simulink model "differential_drive"  (R2023b)
settings: Solver=VariableStepAuto  StartTime=0.0  StopTime=SimulationTime  RelTol=1e-3
values from neighbouring files (symbols this model uses):
  D_ao = 1    [gtg_ao_wf.m]
  D_wf = 1.5    [gtg_ao_wf.m]
  l = 0.5    [gtg_ao_wf.m]
  P = 10    [gtg_ao_wf.m]
  r = 0.1    [gtg_ao_wf.m]
  thetainit = 0    [gtg_ao_wf.m]
  tol = 0.1    [gtg_ao_wf.m]
  v = 0.1    [gtg_ao_wf.m]
  xg = gPos(2)    [gtg_ao_wf.m]
  xinit = sPos(2)    [gtg_ao_wf.m]
  yg = gPos(1)    [gtg_ao_wf.m]
  yinit = sPos(1)    [gtg_ao_wf.m]
undefined symbols (not defined in the file or in its folder): Z
libraries: slpidlib x1
settings Model: PauseTimes=425  PacingRate=0.100000  Creator=npn01  LastModifiedBy=Mikael
settings SolverCC: AlgebraicLoopSolver=TrustRegion
settings DebuggingCC: UnconnectedInputMsg=warning  UnconnectedOutputMsg=warning  UnconnectedLineMsg=warning  ArithmeticOperatorsInVariantConditions=warning
settings ModelReferenceCC: EnableRefExpFcnMdlSchedulingChecks=on
settings SFSimCC: CustomCodeUndefinedFunction=UseInterfaceOnly

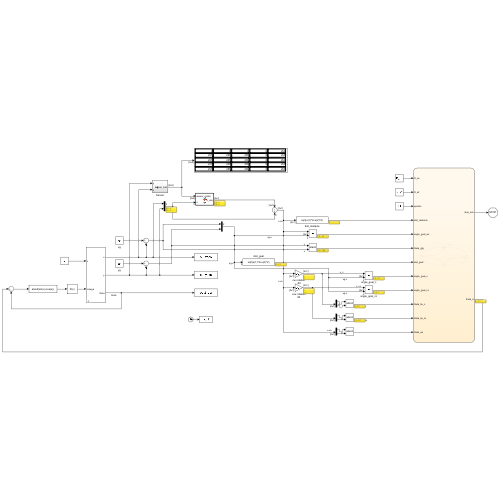
[thumbnail: Simulink's stored preview of the top-level diagram]
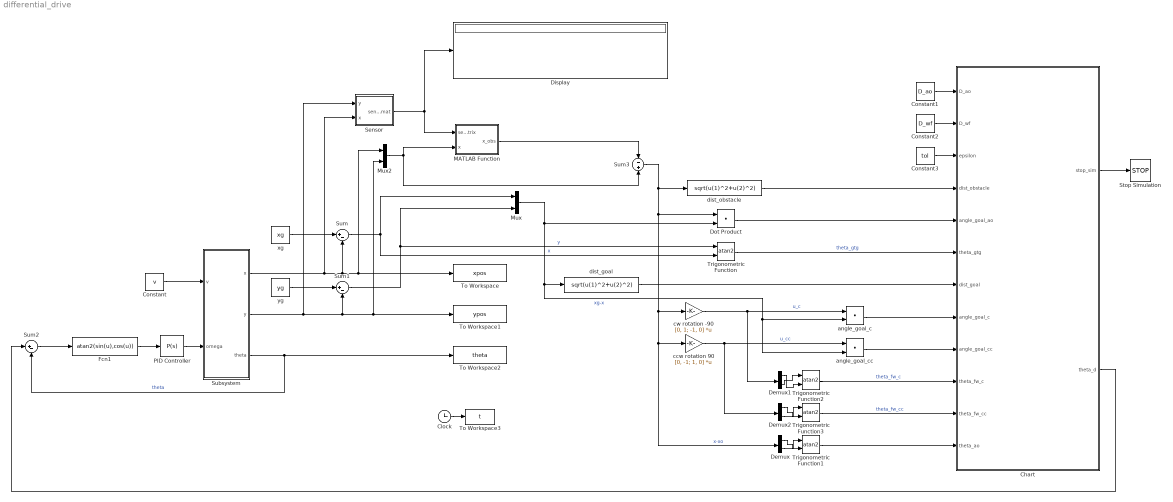
== system differential_drive ==
  Chart : Stateflow chart  TreatAsAtomicUnit=on
  Clock : Clock
  Constant : Constant  Value=v
  Constant1 : Constant  Value=D_ao
  Constant2 : Constant  Value=D_wf
  Constant3 : Constant  Value=tol
  Demux : Demux  Outputs=2
  Demux1 : Demux  Outputs=2
  Demux2 : Demux  Outputs=2
  Display : Display
  Dot Product : DotProduct  OutDataTypeStr=Inherit: Inherit via internal rule
  Fcn1 : Fcn  Expr=atan2(sin(u),cos(u))
  MATLAB Function : MATLAB Function  TreatAsAtomicUnit=on
  Mux : Mux  Inputs=2
  Mux2 : Mux  Inputs=2
  PID Controller : slpidlib/PID Controller  Controller=P  Form=Parallel  TimeDomain=Continuous-time  UseExternalTs=off  SampleTime=-1  IntegratorMethod=Forward Euler  FilterMethod=Forward Euler  ControllerParametersSource=internal  P=P  I=0  UseKiTs=off  D=0  N=100  UseFilter=on  TunerSelectOption=Transfer Function Based (PID Tuner App)  InitialConditionSource=internal  InitialConditionForIntegrator=0  InitialConditionForFilter=0  DifferentiatorICPrevScaledInput=0  ExternalReset=none  TrackingMode=off  Kt=1  LimitOutput=off  SatLimitsSource=internal  UpperSaturationLimit=inf  LowerSaturationLimit=-inf  LinearizeAsGain=on  AntiWindupMode=none  Kb=1  LimitIntegrator=off  UpperIntegratorSaturationLimit=inf  LowerIntegratorSaturationLimit=-inf  POutMin=[]  POutMax=[]  IOutMin=[]  IOutMax=[]  DOutMin=[]  DOutMax=[]  NOutMin=[]  NOutMax=[]  SumOutMin=[]  SumOutMax=[]  SaturationOutMin=[]  SaturationOutMax=[]  PParamMin=[]  PParamMax=[]  IParamMin=[]  IParamMax=[]  DParamMin=[]  DParamMax=[]  NParamMin=[]  NParamMax=[]  KbParamMin=[]  KbParamMax=[]  KtParamMin=[]  KtParamMax=[]  KbOutMin=[]  KbOutMax=[]  KtOutMin=[]  KtOutMax=[]  IntegratorOutMin=[]  IntegratorOutMax=[]  FilterOutMin=[]  FilterOutMax=[]  SumI1OutMin=[]  SumI1OutMax=[]  SumI2OutMin=[]  SumI2OutMax=[]  SumI3OutMin=[]  SumI3OutMax=[]  SumI4OutMin=[]  SumI4OutMax=[]  SumDOutMin=[]  SumDOutMax=[]  DifferentiatorOutMin=[]  DifferentiatorOutMax=[]  FilterDiffOutCoefMin=[]  FilterDiffOutCoefMax=[]  ReciprocalOutMin=[]  ReciprocalOutMax=[]  SumDenOutMin=[]  SumDenOutMax=[]  SumNumOutMin=[]  SumNumOutMax=[]  DivideOutMin=[]  DivideOutMax=[]  UdiffTsProdOutMin=[]  UdiffTsProdOutMax=[]  NTsProdOutMin=[]  NTsProdOutMax=[]  UintegralTsProdOutMin=[]  UintegralTsProdOutMax=[]  UngainTsProdOutMin=[]  UngainTsProdOutMax=[]  ClampingZeroOutDataTypeStr=Inherit: Inherit via back propagation  ClampingZeroOutMin=[]  ClampingZeroOutMax=[]  FilterDenConstantOutDataTypeStr=Inherit: Inherit via back propagation  FilterDenConstantOutMin=[]  FilterDenConstantOutMax=[]  PCopyOutDataTypeStr=Inherit: Inherit via back propagation  PCopyOutMin=[]  PCopyOutMax=[]  NCopyOutDataTypeStr=Inherit: Inherit via back propagation  NCopyOutMin=[]  NCopyOutMax=[]  IntegratorContinuousStateAttributes=''  IntegratorStateMustResolveToSignalObject=off  IntegratorRTWStateStorageClass=Auto  FilterContinuousStateAttributes=''  FilterStateMustResolveToSignalObject=off  FilterRTWStateStorageClass=Auto  ParallelPVariant=InternalParameters  IdealPVariant=Disabled  IVariant=Disabled  DVariant=Disabled  IntegratorVariant=Disabled  SatVariant=Disabled  AWVariant=Disabled  PCopyVariant=Disabled  TRVariant=Disabled  FdbkBlocksVariant=Forward  IdealPFdbkVariant=Disabled  SatFdbkVariant=Disabled  DerivativeFilterVariant=Disabled  NVariant=Disabled  NCopyVariant=Disabled_SignalSpec  FilterICVariant=Disabled  IntegratorICVariant=Disabled  ExternalResetVariant=Disabled  TRSumVariant=Passthrough  SumFdbkVariant=Disabled  SumVariant=Passthrough_P  TsampFilterVariant=InternalTs  TsampNgainVariant=Passthrough  TsampIntegralVariant=Disabled_SignalSpec  ExternalSaturationOutDataTypeStr=Inherit: Same as second input
  Sensor : Subsystem
  Stop Simulation : Stop
  Subsystem : Subsystem  mask{x0=xinit, y0=yinit, theta0=thetainit}
      mask DialogControl Control4 Prompt: Enter x initial position
      mask DialogControl Control2 Prompt: Enter y initial position
      mask DialogControl Control3 Prompt: Enter initial theta angle
      mask DialogControl Control6 Prompt: Any text you want
  Sum : Sum  Inputs=|+-
  Sum1 : Sum  Inputs=|+-
  Sum2 : Sum  Inputs=|+-
  Sum3 : Sum  Inputs=-+
  To Workspace : ToWorkspace  VariableName=xpos  SampleTime=-1
  To Workspace1 : ToWorkspace  VariableName=ypos  SampleTime=-1
  To Workspace2 : ToWorkspace  VariableName=theta  SampleTime=-1
  To Workspace3 : ToWorkspace  VariableName=t  SampleTime=-1
      settings: Save2DSignal=2-D array (concatenate along first dimension)
  Trigonometric Function{,1..3} (4 alike) : Trigonometry  Operator=atan2
  angle_goal_c : DotProduct  OutDataTypeStr=Inherit: Inherit via internal rule
  angle_goal_cc : DotProduct  OutDataTypeStr=Inherit: Inherit via internal rule
  ccw rotation 90 : Gain  Gain=[0, -1; 1, 0]  Multiplication=Matrix(K*u)
  cw rotation -90 : Gain  Gain=[0, 1; -1, 0]  Multiplication=Matrix(K*u)
  dist_goal : Fcn  Expr=sqrt(u(1)^2+u(2)^2)
  dist_obstacle : Fcn  Expr=sqrt(u(1)^2+u(2)^2)
  xg : Constant  Value=xg
  yg : Constant  Value=yg
  wires:
  Constant/1 -> Subsystem/1(v)
  xg/1 -> Sum/1
  Subsystem/1(x) -> Sensor/2(x), Mux2/1, To Workspace/1, Sum/2
  yg/1 -> Sum1/1
  Subsystem/2(y) -> Sensor/1(y), Sum1/2, Mux2/2, To Workspace1/1
  Sum/1 -> Trigonometric Function/2, Mux/1  "x"
  Subsystem/3(theta) -> To Workspace2/1, Sum2/2  "theta"
  PID Controller/1 -> Subsystem/2(omega)
  Sum2/1 -> Fcn1/1
  Fcn1/1 -> PID Controller/1
  Clock/1 -> To Workspace3/1
  Mux/1 -> angle_goal_cc/2, angle_goal_c/2, dist_goal/1, Dot Product/2  "xg-x"
  Sum1/1 -> Mux/2, Trigonometric Function/1  "y"
  Mux2/1 -> MATLAB Function/2(x), Sum3/2
  Sum3/1 -> Demux/1, ccw rotation 90/1, cw rotation -90/1, Dot Product/1, dist_obstacle/1  "x-xo"
  cw rotation -90/1 -> angle_goal_c/1, Demux1/1  "u_c"
  ccw rotation 90/1 -> angle_goal_cc/1, Demux2/1  "u_cc"
  Trigonometric Function/1 -> Chart/6(theta_gtg)  "theta_gtg"
  Chart/1(stop_sim) -> Stop Simulation/1
  Chart/2(theta_d) -> Sum2/1
  dist_goal/1 -> Chart/7(dist_goal)
  dist_obstacle/1 -> Chart/4(dist_obstacle)
  Constant3/1 -> Chart/3(epsilon)
  Constant2/1 -> Chart/2(D_wf)
  Constant1/1 -> Chart/1(D_ao)
  angle_goal_c/1 -> Chart/8(angle_goal_c)
  angle_goal_cc/1 -> Chart/9(angle_goal_cc)
  Dot Product/1 -> Chart/5(angle_goal_ao)
  Trigonometric Function2/1 -> Chart/10(theta_fw_c)  "theta_fw_c"
  Trigonometric Function3/1 -> Chart/11(theta_fw_cc)  "theta_fw_cc"
  Demux/1 -> Trigonometric Function1/2
  Demux/2 -> Trigonometric Function1/1
  Demux1/1 -> Trigonometric Function2/2
  Demux1/2 -> Trigonometric Function2/1
  Demux2/1 -> Trigonometric Function3/2
  Demux2/2 -> Trigonometric Function3/1
  Sensor/1(sensor_mat) -> Display/1, MATLAB Function/1(sensor_matrix)
  MATLAB Function/1(x_obs) -> Sum3/1
  Trigonometric Function1/1 -> Chart/12(theta_ao)

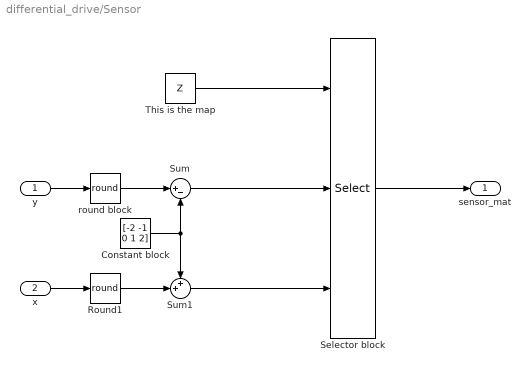
== system differential_drive/Sensor ==
  y : Inport
  x : Inport  Port=2
  Constant block : Constant  Value=[-2 -1 0 1 2]
  Round1 : Rounding  Operator=round
  Selector block : Selector  NumberOfDimensions=2  InputPortWidth=3  IndexOptions=Index vector (port),Index vector (port)  Indices=[1 3],1  OutputSizes=1,1
  Sum : Sum  Inputs=|+-  OutDataTypeStr=int32  RndMeth=Round
  Sum1 : Sum  Inputs=++|  OutDataTypeStr=int32  RndMeth=Round
  This is the map : Constant  Value=Z  VectorParams1D=off
  round block : Rounding  Operator=round
  sensor_mat : Outport
  wires:
  This is the map/1 -> Selector block/1
  Constant block/1 -> Sum1/1, Sum/2
  Sum/1 -> Selector block/2
  Sum1/1 -> Selector block/3
  Selector block/1 -> sensor_mat/1
  y/1 -> round block/1
  round block/1 -> Sum/1
  x/1 -> Round1/1
  Round1/1 -> Sum1/2

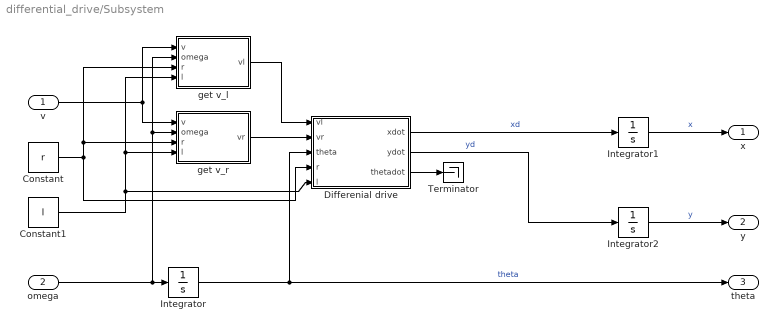
== system differential_drive/Subsystem ==
  v : Inport
  omega : Inport  Port=2
  Constant : Constant  Value=r
  Constant1 : Constant  Value=l
  Differenial drive : MATLAB Function  TreatAsAtomicUnit=on
  Integrator : Integrator  InitialCondition=theta0
  Integrator1 : Integrator  InitialCondition=x0
  Integrator2 : Integrator  InitialCondition=y0
  Terminator : Terminator
  get v_l : MATLAB Function  TreatAsAtomicUnit=on
  get v_r : MATLAB Function  TreatAsAtomicUnit=on
  x : Outport
  y : Outport  Port=2
  theta : Outport  Port=3
  wires:
  Differenial drive/2(ydot) -> Integrator2/1  "yd"
  Integrator2/1 -> y/1  "y"
  Integrator/1 -> Differenial drive/3(theta), theta/1  "theta"
  Differenial drive/1(xdot) -> Integrator1/1  "xd"
  omega/1 -> get v_l/2(omega), get v_r/2(omega), Integrator/1
  Integrator1/1 -> x/1  "x"
  v/1 -> get v_r/1(v), get v_l/1(v)
  get v_l/1(vl) -> Differenial drive/1(vl)
  get v_r/1(vr) -> Differenial drive/2(vr)
  Constant/1 -> get v_r/3(r), get v_l/3(r), Differenial drive/4(r)
  Constant1/1 -> get v_l/4(l), get v_r/4(l), Differenial drive/5(l)
  Differenial drive/3(thetadot) -> Terminator/1

== matlab function differential_drive/Subsystem/get v_r ==
  data: v input; vr output; omega input; r input; l input
function vr = fcn(v, omega, r, l)

vr = get_vr(v, omega, r, l);

== matlab function differential_drive/Subsystem/get v_l ==
  data: v input; vl output; omega input; r input; l input
function vl = fcn(v, omega, r, l)

vl = get_vl(v, omega, r, l);

== matlab function differential_drive/Subsystem/Differenial drive ==
  data: vl input; xdot output; vr input; theta input; r input; l input; ydot output; thetadot output
function [xdot, ydot, thetadot] = fcn(vl, vr, theta, r, l)

[xdot, ydot, thetadot] = differential_drive_xytheta(vl, vr, theta, r, l);

== matlab function differential_drive/MATLAB Function ==
  data: sensor_matrix input; x_obs output; x input
function x_obs = fcn(sensor_matrix, x)

x_obs = find_obs(sensor_matrix, x);

== stateflow chart differential_drive/Chart ==
  state S_stop
    entry:
    stop_sim = 1;
  state S_GTG
    during:
    theta_d = theta_gtg;
  state S_FW_CC
    during:
    theta_d = theta_fw_cc;
  state S_FW_C
    during:
    theta_d = theta_fw_c;
  state S_AO
    during:
    theta_d = theta_ao;
  (default) -> S_GTG : {stop_sim = 0;
      | theta_d = 0;
      | }
  S_GTG -> S_stop [order 3] : [dist_goal < epsilon]
  S_GTG -> S_FW_C [order 2] : [(dist_obstacle < D_wf) && (angle_goal_c > 0)]{d_tau = dist_goal;}
  S_GTG -> S_FW_CC [order 1] : [(dist_obstacle < D_wf) && (angle_goal_cc > 0)]{d_tau = dist_goal;}
  S_FW_CC -> S_GTG [order 2] : [(dist_goal < d_tau) && (angle_goal_ao > 0)]
  S_FW_C -> S_GTG [order 2] : [(dist_goal < d_tau) && (angle_goal_ao > 0)]
  S_AO -> S_FW_CC [order 2] : [(dist_obstacle >= D_ao) && (angle_goal_cc > 0)]{d_tau = dist_goal;}
  S_AO -> S_FW_C [order 1] : [(dist_obstacle >= D_ao) && (angle_goal_c > 0)]{d_tau = dist_goal;}
  S_FW_CC -> S_AO [order 1] : [dist_obstacle < D_ao]
  S_FW_C -> S_AO [order 1] : [dist_obstacle < D_ao]
  data: D_ao input; D_wf input; epsilon input; dist_obstacle input; d_tau local; stop_sim output; theta_d output; angle_goal_ao input; theta_gtg input; dist_goal input; angle_goal_c input; angle_goal_cc input; theta_fw_c input; theta_fw_cc input; theta_ao input
